simulink model "slexMultiInstanceFunctionsExample_org"  (Simulink 10.0)
settings: Solver=FixedStepDiscrete  StartTime=0.0  StopTime=100  FixedStep=0.1  RelTol=1e-3
InitFcn:
  | warning('off','Simulink:Logging:DatasetRTWGenRootOutputNotSupported');
  | warning('off','Simulink:Logging:DatasetRTWGenStateNotSupported');
StartFcn:
  | warning('off','Simulink:Logging:DatasetRTWGenRootOutputNotSupported');
  | warning('off','Simulink:Logging:DatasetRTWGenStateNotSupported');
StopFcn:
  | warning('on','Simulink:Logging:DatasetRTWGenRootOutputNotSupported');
  | warning('on','Simulink:Logging:DatasetRTWGenStateNotSupported');
CloseFcn:
  | warning('on','Simulink:Logging:DatasetRTWGenRootOutputNotSupported');
  | warning('on','Simulink:Logging:DatasetRTWGenStateNotSupported');
PauseFcn:
  | warning('on','Simulink:Logging:DatasetRTWGenRootOutputNotSupported');
  | warning('on','Simulink:Logging:DatasetRTWGenStateNotSupported');
settings Model: Creator=The MathWorks, Inc.  ModifiedByFormat=The MathWorks Inc.  LastModifiedBy=The MathWorks Inc.  ExtModeAutoUpdateStatusClock=off
settings DataIOCC: LimitDataPoints=on  SaveFinalState=on  SaveState=on  ReturnWorkspaceOutputs=on  SignalLoggingName=logsOut
settings OptimizationCC: DefaultParameterBehavior=Inlined  InlineInvariantSignals=on  PassReuseOutputArgsAs=Individual arguments  ExpressionDepthLimit=2147483647  InitFltsAndDblsToZero=on  LifeSpan=auto  EfficientTunableParamExpr=on
settings DebuggingCC: SaveWithParameterizedLinksMsg=none  UnderspecifiedInitializationDetection=Simplified  MergeDetectMultiDrivingBlocksExec=error  CheckExecutionContextPreStartOutputMsg=on  CheckExecutionContextRuntimeOutputMsg=on  MultiTaskDSMMsg=warning  MultiTaskCondExecSysMsg=none  SigSpecEnsureSampleTimeMsg=none  ParameterTunabilityLossMsg=error  FcnCallInpInsideContextMsg=warning  AllowSymbolicDim=off  StateNameClashWarn=warning  StrictBusMsg=ErrorOnBusTreatedAsVector
settings HardwareCC: TargetHWDeviceType=32-bit Generic
settings ModelReferenceCC: UpdateModelReferenceTargets=IfOutOfDate  CheckModelReferenceTargetMessage=none
settings SFSimCC: MATLABDynamicMemAlloc=off
settings RTWCC: Description=Embedded Coder  SystemTargetFile=ert.tlc  TemplateMakefile=ert_default_tmf  GenerateReport=on  IncludeHyperlinkInReport=on  LaunchReport=on  GenerateTraceInfo=on  GenerateTraceReport=on  GenerateTraceReportSl=on  GenerateTraceReportSf=on  GenerateTraceReportEml=on
settings CodeAppCC: ForceParamTrailComments=on  IgnoreCustomStorageClasses=off  MaxIdLength=100  OperatorAnnotations=on  SimulinkDataObjDesc=on  SFDataObjDesc=on  InsertBlockDesc=on  StateflowObjectComments=off
settings ERTTargetCC: GenerateSampleERTMain=on  InlinedParameterPlacement=NonHierarchical  ERTCustomFileTemplate=example_file_process.tlc
settings ConfigComp: CovExternalEMLEnable=off  CovSFcnEnable=off

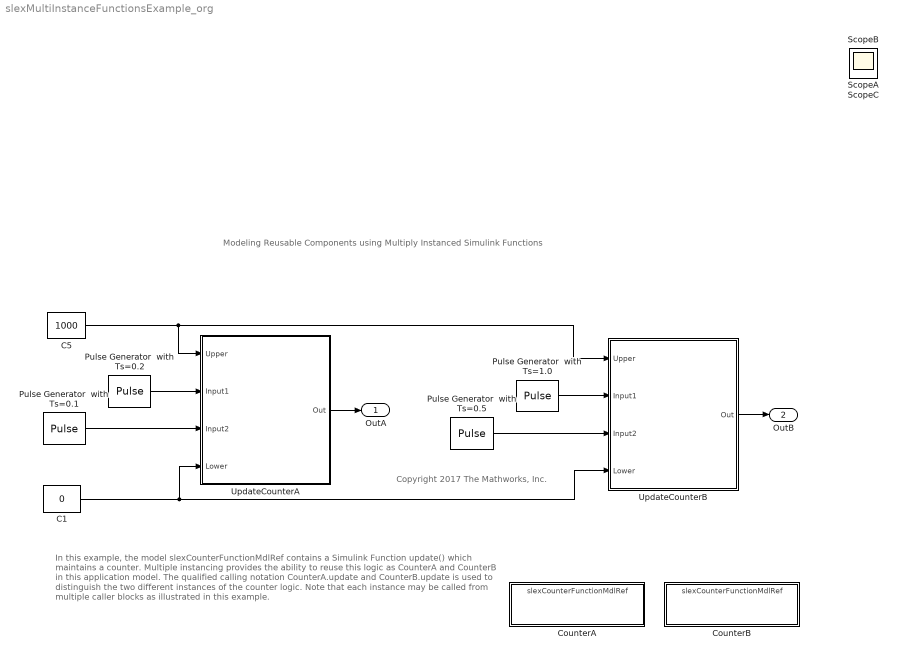
== system slexMultiInstanceFunctionsExample_org ==
  note: Modeling Reusable Components
      | using Multiply Instanced Simulink Functions
  note: Copyright 2017 The Mathworks, Inc.
  note: In this example, the model slexCounterFunctionMdlRef contains a Simulink Function update() which maintains a counter. Multiple instancing provides the ability to reuse this logic as CounterA and CounterB in this application model.
      |
      | The qualified calling notation CounterA.update and CounterB.update is used to distinguish the two different instances of the counter logic. Note that each instance may be called from multiple caller blocks as illustrated in this example.
  C1 : Constant  Value=0
  C5 : Constant  Value=1000
  CounterA : ModelReference  ModelNameDialog=slexCounterFunctionMdlRef.slx  SimulationMode=Normal  ScheduleRates=on  ModelReferenceVersion=1.88
  CounterB : ModelReference  ModelNameDialog=slexCounterFunctionMdlRef.slx  SimulationMode=Normal  ScheduleRates=on  ModelReferenceVersion=1.88
  Pulse Generator  with Ts=0.1 : DiscretePulseGenerator  SampleTime=0.1  VectorParams1D=off
  Pulse Generator  with Ts=0.2 : DiscretePulseGenerator  SampleTime=0.2  VectorParams1D=off
  Pulse Generator  with Ts=0.5 : DiscretePulseGenerator  SampleTime=0.5
  Pulse Generator  with Ts=1.0 : DiscretePulseGenerator
  UpdateCounterA : Subsystem
  UpdateCounterB : Subsystem
  OutA : Outport  VectorParamsAs1DForOutWhenUnconnected=off
  OutB : Outport  Port=2  VectorParamsAs1DForOutWhenUnconnected=off
  ScopeA : Scope
  ScopeB : Scope
  ScopeC : Scope
  wires:
  C1/1 -> UpdateCounterB/4(Lower), UpdateCounterA/4(Lower)
  C5/1 -> UpdateCounterB/1(Upper), UpdateCounterA/1(Upper)
  UpdateCounterB/1(Out) -> OutB/1
  Pulse Generator  with Ts=0.2/1 -> UpdateCounterA/2(Input1)
  Pulse Generator  with Ts=1.0/1 -> UpdateCounterB/2(Input1)
  Pulse Generator  with Ts=0.5/1 -> UpdateCounterB/3(Input2)
  UpdateCounterA/1(Out) -> OutA/1
  Pulse Generator  with Ts=0.1/1 -> UpdateCounterA/3(Input2)

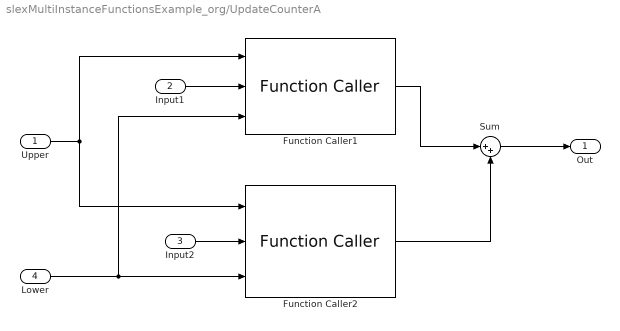
== system slexMultiInstanceFunctionsExample_org/UpdateCounterA ==
  Upper : Inport
  Input1 : Inport  Port=2
  Input2 : Inport  Port=3
  Lower : Inport  Port=4
  Function Caller1 : FunctionCaller  FunctionPrototype=output = CounterA.update(upper,input,lower)  InputArgumentSpecifications=<Enter example>  OutputArgumentSpecifications=<Enter example>
  Function Caller2 : FunctionCaller  FunctionPrototype=output = CounterA.update(upper,input,lower)  InputArgumentSpecifications=<Enter example>  OutputArgumentSpecifications=<Enter example>
  Sum : Sum  Inputs=|++
  Out : Outport  VectorParamsAs1DForOutWhenUnconnected=off
  wires:
  Function Caller1/1 -> Sum/1
  Upper/1 -> Function Caller2/1, Function Caller1/1
  Function Caller2/1 -> Sum/2
  Input2/1 -> Function Caller2/2
  Sum/1 -> Out/1
  Input1/1 -> Function Caller1/2
  Lower/1 -> Function Caller1/3, Function Caller2/3

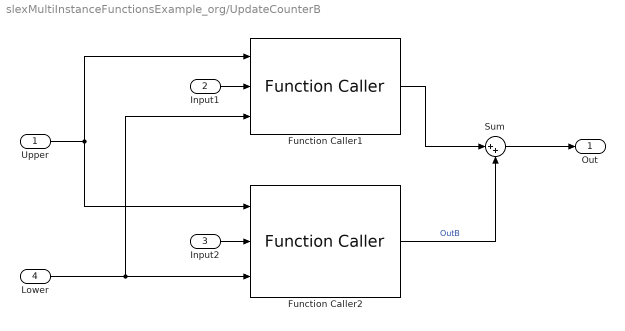
== system slexMultiInstanceFunctionsExample_org/UpdateCounterB ==
  Upper : Inport
  Input1 : Inport  Port=2
  Input2 : Inport  Port=3
  Lower : Inport  Port=4
  Function Caller1 : FunctionCaller  FunctionPrototype=output = CounterB.update(upper,input,lower)  InputArgumentSpecifications=<Enter example>  OutputArgumentSpecifications=<Enter example>
  Function Caller2 : FunctionCaller  FunctionPrototype=output = CounterB.update(upper,input,lower)  InputArgumentSpecifications=<Enter example>  OutputArgumentSpecifications=<Enter example>
  Sum : Sum  Inputs=|++
  Out : Outport  VectorParamsAs1DForOutWhenUnconnected=off
  wires:
  Upper/1 -> Function Caller2/1, Function Caller1/1
  Input2/1 -> Function Caller2/2
  Lower/1 -> Function Caller1/3, Function Caller2/3
  Input1/1 -> Function Caller1/2
  Function Caller1/1 -> Sum/1
  Function Caller2/1 -> Sum/2  "OutB"
  Sum/1 -> Out/1
